simulink model "c1"  (R2021b)
settings: Solver=VariableStepAuto  StartTime=0.0  StopTime=10.0  RelTol=1e-3
settings Model: Creator=asus  LastModifiedBy=Newsky

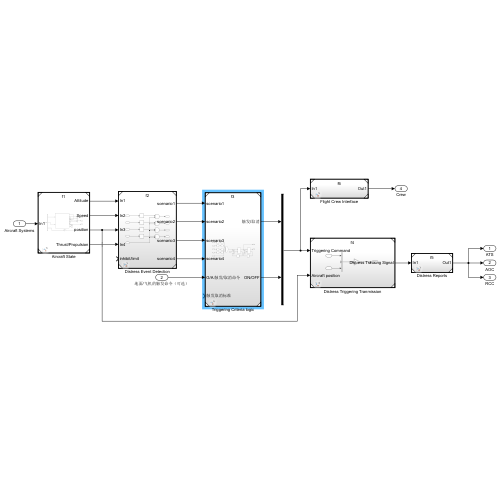
[thumbnail: Simulink's stored preview of the top-level diagram]
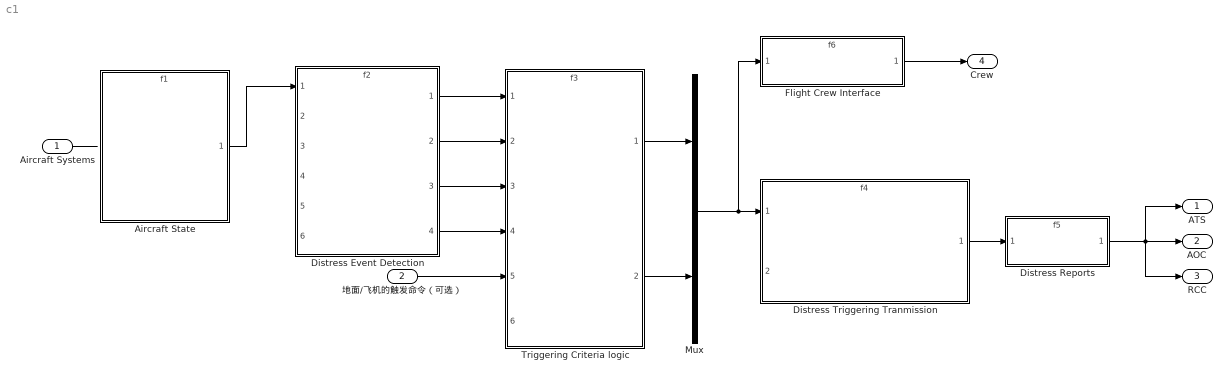
== system c1 ==
  Aircraft Systems : Inport
  地面/飞机的触发命令（可选） : Inport  Port=2
  Aircraft State : ModelReference  ModelNameDialog=f1.slx  SimulationMode=Normal  ModelReferenceVersion=1.12
  Distress Event Detection : ModelReference  ModelNameDialog=f2.slx  SimulationMode=Normal  ModelReferenceVersion=1.10
  Distress Reports : ModelReference  ModelNameDialog=f5.slx  SimulationMode=Normal  ModelReferenceVersion=1.1
  Distress Triggering Tranmission : ModelReference  ModelNameDialog=f4.slx  SimulationMode=Normal  ModelReferenceVersion=1.6
  Flight Crew Interface : ModelReference  ModelNameDialog=f6.slx  SimulationMode=Normal  ModelReferenceVersion=1.1
  Mux : Mux  Inputs=2
  Triggering Criteria logic : ModelReference  ModelNameDialog=f3.slx  SimulationMode=Normal  ModelReferenceVersion=1.21
  ATS : Outport
  AOC : Outport  Port=2
  RCC : Outport  Port=3
  Crew : Outport  Port=4
  wires:
  Aircraft State/1 -> Distress Event Detection/1
  ? -> Distress Event Detection/2
  ? -> Distress Triggering Tranmission/2, Distress Event Detection/3
  ? -> Distress Event Detection/4
  Distress Event Detection/1 -> Triggering Criteria logic/1
  Distress Event Detection/2 -> Triggering Criteria logic/2
  Distress Event Detection/3 -> Triggering Criteria logic/3
  Distress Event Detection/4 -> Triggering Criteria logic/4
  Aircraft Systems/1 -> ?
  地面/飞机的触发命令（可选）/1 -> Triggering Criteria logic/5
  Triggering Criteria logic/1 -> Mux/1
  Triggering Criteria logic/2 -> Mux/2
  Mux/1 -> Flight Crew Interface/1, Distress Triggering Tranmission/1
  Distress Triggering Tranmission/1 -> Distress Reports/1
  Distress Reports/1 -> RCC/1, AOC/1, ATS/1
  Flight Crew Interface/1 -> Crew/1
